simulink model "f"  (R2019a)
settings: Solver=VariableStepAuto  StartTime=0.0  StopTime=10.0  RelTol=1e-3
settings Model: Creator=rache  LastModifiedBy=rache
settings DataIOCC: ReturnWorkspaceOutputs=off
settings DebuggingCC: ArithmeticOperatorsInVariantConditions=warning

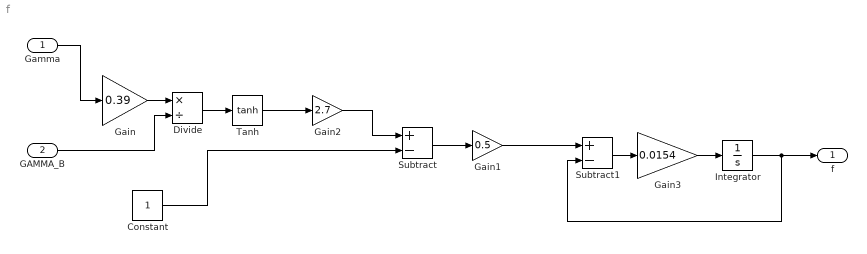
== system f ==
  Gamma : Inport
  GAMMA_B : Inport  Port=2
  Constant : Constant
  Divide : Product  Inputs=*/
  Gain : Gain  Gain=0.39
  Gain1 : Gain  Gain=0.5
  Gain2 : Gain  Gain=2.7
  Gain3 : Gain  Gain=0.0154
  Integrator : Integrator
  Subtract : Sum  Inputs=+-
  Subtract1 : Sum  Inputs=+-
  Tanh : Trigonometry  Operator=tanh
  f : Outport
  wires:
  Integrator/1 -> Subtract1/2, f/1
  Gamma/1 -> Gain/1
  Gain/1 -> Divide/1
  GAMMA_B/1 -> Divide/2
  Constant/1 -> Subtract/2
  Subtract/1 -> Gain1/1
  Divide/1 -> Tanh/1
  Tanh/1 -> Gain2/1
  Gain2/1 -> Subtract/1
  Gain1/1 -> Subtract1/1
  Subtract1/1 -> Gain3/1
  Gain3/1 -> Integrator/1
